simulink model "Drone2_simulink"  (R2024a)
settings: Solver=ode1be  StartTime=0.0  StopTime=1000  FixedStep=0.001  MaxStep=0.001  MinStep=0.00095  RelTol=1e-3
PreLoadFcn:
  | Drone_data;
model workspace: external: MATLAB File C:\Users\admin\OneDrive - Indian Institute of Technology Jodhpur\IIT JODHPUR\Research Work\Amphibious Drone\MATLAB_CODE\2025\New_Drone\Drone_1\Drone1_simulink_DataFile.m (data not in the file)
undefined symbols (not defined in the file): Environment, Newton, Raphson, Vehicle, X, Y, Z
libraries: sm_lib x1684, nesl_utility x63, slpidlib x25, eeGeneralControl x6, matrix_library x3, rllib x2, simulink x2, fl_lib x1, sharedutil x1, SignalEditorBlockLib x1
(part 17 of 17)

== matlab function Drone2_simulink/Controller1/Underwater_Syringe_Actuation/MATLAB Function7 ==
  settings: updateMethod=DISCRETE
  data: Z_desired input; Z input; F_b input; tb input; Vf_cmd output; ez input; ez_dot input; etheta input; etheta_dot input; Vb_cmd output; Vf_prev input; Vb_prev input; Vf_trim_hat output; Vb_trim_hat output; Max parameter; Min parameter; DFRate parameter; DMRate parameter; DSRate parameter; Dpanelty parameter; EZDB parameter; PLRate parameter; PKRate parameter; ETDB parameter; RHO parameter; G parameter; AS parameter; HF parameter; DT parameter
function [Vf_cmd, Vb_cmd, Vf_trim_hat, Vb_trim_hat]= ...
    syringe_allocation_adaptive(Z_desired, Z,F_b,tb, ez, ez_dot,etheta,etheta_dot,Vf_prev, Vb_prev,Max, Min,DFRate, DMRate, DSRate, Dpanelty, EZDB, PLRate, PKRate, ETDB,RHO, G,AS,HF,DT)
% Depth-only allocator with adaptive trims for 2 front syringes (identical) + 1 rear.
% Units: meters of stroke for all volumes/positions.
% Outputs:
%   Vf_cmd       -> per-front syringe command (send same to both fronts)
%   Vb_cmd       -> rear syringe command
%   Vf_trim_hat  -> current estimated per-front trim (for datalogging/observability)
%   Vb_trim_hat  -> current estimated rear trim

% -------- Tunables --------
rho = RHO; %1000;         % kg/m^3
g   = G; %9.81;         % m/s^2
A   = AS; %0.026;        % m^2  (verify; adjust to your syringe)
l= HF; %0.2;
V_MIN = Min;      % m (5 mm)
V_MAX = Max;      % m (100 mm)
V_DOT_MAX = 0.012;  % m/s (12 mm/s)
dt = DT; %0.001;
tb = clamp(tb,-5,5);

% -------- Persistent state for trim estimates --------
persistent VF_TRIM VF_TRIM_INIT VB_TRIM VB_TRIM_INIT inited
if isempty(inited)
    VF_TRIM_INIT = 0.046;   % m  (assumed 46 mm per front syringe)
    VB_TRIM_INIT = 0.031;   % m  (assumed 31 mm rear syringe)
    VF_TRIM = VF_TRIM_INIT;
    VB_TRIM = VB_TRIM_INIT;
    inited = true;
end


if Z_desired >-0.1 || Z>=0
    Vf_cmd = Min;
    Vb_cmd = Min;
    Vf_trim_hat = Vf_cmd;
    Vb_trim_hat = Vb_cmd;
    return
end


persistent t
if isempty(t)
    t =0;
end

% S = 2*Vf_prev+Vb_prev;
 % kp =0;
% Adaptive-trim gains (start small)
if abs(ez) > 1
    K_TRIM_eff = DFRate;%0.02;   % fast learning when far
    kp = 0;
elseif abs(ez) > 0.6
    K_TRIM_eff = DMRate; %0.005;   % medium
    kp= 0;
else
    K_TRIM_eff = DSRate; %0.002;  % fine adjust near trim
    if abs(ez)<0.2
        t=t+1;
    else
        t = 0;
    end
    if t>50000
        kp=1;
    else
        kp =0;
    end

end


K_TRIM  =K_TRIM_eff;    % (m/s per m of depth error)  VERY SLOW 0.002
K_RATE  = Dpanelty; %0.05;     % dimensionless; reduces adaptation if |ez_dot| is large 0.05
EZ_DB   = EZDB; %0.05;     % m; within 10 cm, adapt 5x slower to avoid chatter 0.05

KP_TRIM  =PLRate; %0.0002;    % (m/s per m of depth error)  VERY SLOW 0.002
K_Pitch_Rate  = PKRate; %0.05;     % dimensionless; reduces adaptation if |ez_dot| is large 0.05
Etheta_DB   = deg2rad(ETDB); %pi/60;     % m; within 10 cm, adapt 5x slower to avoid chatter 0.05




% -------- Fast (reactive) path from F_b to stroke increments --------
% F_b = rho*g*A*(2*Vf_inc + Vb_inc)
dSum = F_b / (rho*g*A);   % meters of stroke-sum (2*Vf + Vb)
Vf_inc_fast = 0.25 * dSum;  % per front syringe
Vb_inc_fast = 0.50 * dSum;  % rear


%-------- Pitch Control-----
mSum = tb/(rho*g*A*l);
%mSum = tb/(rho*g*A*(2*(l-0.5*Vf_prev)-(l-0.5*Vb_prev)));
%mSum = (tb-rho*A*g*S*(l-0.5*Vf_prev))/(rho*g*A*(2*(l-0.5*Vf_prev)-(l-0.5*Vb_prev)));
Vf_inc_pitch = 0.5*mSum;
vb_inc_pitch = -0.5*mSum;
Vf_inc_pitch = clamp(Vf_inc_pitch,-0.005,0.005);
vb_inc_pitch = clamp(vb_inc_pitch,-0.01,0.01);


% -------- Slow (adaptive) trim update to remove drift --------
% adapt_gate = exp(-K_RATE*abs(ez_dot));

adapt_gate = 1.0 / (1.0 + K_RATE*abs(ez_dot));     % suppress when moving fast
if abs(ez) < EZ_DB
    adapt_gate = 0.25 * adapt_gate;                 % slower inside small band0.2
end
dSum_trim = K_TRIM * ez * adapt_gate;              % m/s equivalent stroke-sum


%------ Pitch updates

pitch_gate = kp/(1.0+K_Pitch_Rate*abs(etheta_dot));
if abs(etheta) <Etheta_DB
    pitch_gate = 0.2*pitch_gate;
end
mSum_trim = KP_TRIM*etheta*pitch_gate;
mSum_trim = clamp(mSum_trim,-0.01,0.01);


Vf_trim_update = 0.25 * dSum_trim * dt-0.25*mSum_trim*dt;            % per front syringe
Vb_trim_update = 0.50 * dSum_trim * dt+0.50*mSum_trim*dt;            % rear

VF_TRIM = clamp(VF_TRIM + Vf_trim_update, V_MIN, V_MAX);
VB_TRIM = clamp(VB_TRIM + Vb_trim_update, V_MIN, V_MAX);

% -------- Combine trim + fast correction --------
Vf_target = VF_TRIM + Vf_inc_fast+0*kp*Vf_inc_pitch;
Vb_target = VB_TRIM + Vb_inc_fast+0*kp*vb_inc_pitch;

% -------- Stroke clamp --------
Vf_target = clamp(Vf_target, V_MIN, V_MAX);
Vb_target = clamp(Vb_target, V_MIN, V_MAX);
Vf_cmd = Vf_target;
Vb_cmd = Vb_target;
% % -------- Rate limit (12 mm/s) --------
% Vf_cmd = rate_limit(Vf_target, Vf_prev, V_DOT_MAX, dt);
% Vb_cmd = rate_limit(Vb_target, Vb_prev, V_DOT_MAX, dt);

% Expose trims for logging/next block
Vf_trim_hat = VF_TRIM;
Vb_trim_hat = VB_TRIM;

end

% ===== helpers =====
function y = clamp(x, xmin, xmax)
    y = min(max(x, xmin), xmax);
end

% function y = rate_limit(cmd, prev, vdot_max, dt)
%     max_step = vdot_max * max(dt,1e-4);
%     y = clamp(cmd, prev - max_step, prev + max_step);
% end

== matlab function Drone2_simulink/Hydrostatic & Hydrodynamic Effects/Buoyancy Force/MATLAB Function ==
  data: Z input; Factor output; a input; b input; y_a input; y_b input; reverse input
function Factor = quadratic_map(Z, a, b, y_a, y_b, reverse)
    % Quadratic mapping from [a, b] to [y_a, y_b]
    % reverse = 0 -> Normal mapping (a -> y_a, b -> y_b)
    % reverse = 1 -> Reverse mapping (a -> y_b, b -> y_a)
    
    c = (y_b - y_a) / (b - a)^2;
    
    if reverse
        Factor = y_b - c * (Z - a).^2;
    else
        Factor = c * (Z - a).^2 + y_a;
    end
end

== matlab function Drone2_simulink/Hydrostatic & Hydrodynamic Effects/Wind force/wind_disturbance ==
  settings: updateMethod=DISCRETE
  data: t input; vx output; v_mean input; v_max input; vy output; vz output
function [vx, vy, vz] = windVelocity(t,v_mean,v_max)
% Deterministic wind with stochastic component
 % mean wind in x
v_turb = 0.5 * sin(0.1 * t) .* randn(3,1);  % small gusts
v_wind = v_mean + v_turb;

% Optionally clamp:
if norm(v_wind) > v_max
    v_wind = 3 * v_wind / norm(v_wind);
end
vx = v_wind(1);
vy = v_wind(2);
vz = v_wind(3);
end

== matlab function Drone2_simulink/Hydrostatic & Hydrodynamic Effects/Ocean Current/MATLAB Function1 ==
  data: t input double size=1; u output double size=1; z input double size=1; maxVel input; v output; w output; MATFile input
function [u, v, w]  = jonswapVelocity(t, z,maxVel,MATFile)
    persistent a omega k phi h theta
    if isempty(a)
        %params = Environment.OceanCurrentFile;
        a = MATFile.a;
        omega = MATFile.omega;
        k = MATFile.k;
        phi = MATFile.phi;
        h = MATFile.h;
        theta = MATFile.theta;
    end

    u = 0;
    v = 0;
    w = 0;

    for i = 1:length(a)
        wi = omega(i);
        ki = k(i);
        phi_i = phi(i);
        th = theta(i);
        denominator = sinh(k(i)*h);
        if abs(denominator) < 1e-8
           denominator = sign(denominator)*1e-8; % avoid zero division
        end

        scale_h = a(i) * wi * cosh(ki * (z + h)) / denominator;
        scale_v = a(i) * wi * sinh(ki * (z + h)) / denominator;

        phase = -wi * t + phi_i;

        u = u + scale_h * cos(th) * cos(phase);
        v = v + scale_h * sin(th) * cos(phase);
        w = w + scale_v * sin(phase);
    end

    % Optional: limit velocity magnitude here if needed
    mag = sqrt(u.^2 + v.^2 + w.^2);
    if mag > maxVel
        scale = maxVel / mag;
        u = u * scale;
        v = v * scale;
        w = w * scale;
    end
    %V_rel = [u;v;w];
end

== matlab function Drone2_simulink/Controller/MATLAB Function ==
  data: Forwardthrust input; l output; yaw input; r output
function [l,r] = fcn(Forwardthrust,yaw)
A=[1 1;-1 1]\[Forwardthrust;yaw];
l = A(1);
r = A(2);
